simulink model "manipuladores_practica_5"  (R2024b)
settings: Solver=VariableStepAuto  StartTime=0.0  StopTime=10  RelTol=1e-3
settings Model: Creator=alema  LastModifiedBy=alema

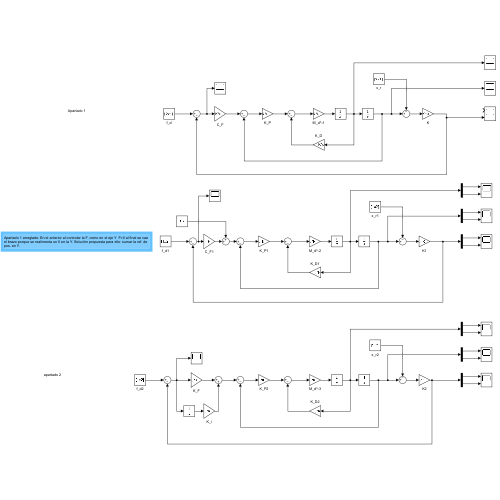
[thumbnail: Simulink's stored preview of the top-level diagram]
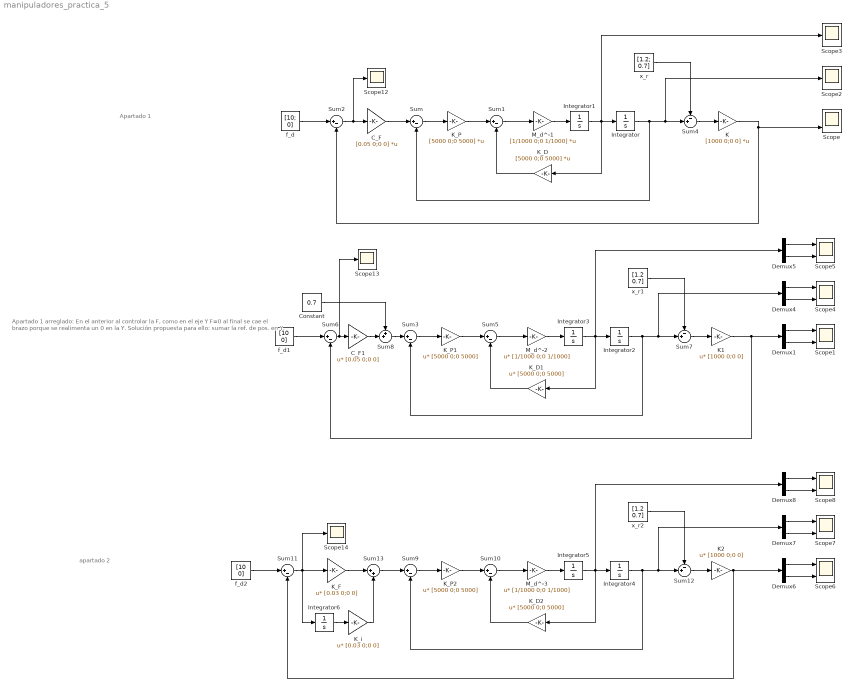
== system manipuladores_practica_5 ==
  note: Apartado 1
  note: Apartado 1 arreglado: En el anterior al controlar la F, como en el eje Y F=0 al final se cae el brazo porque se realimenta un 0 en la Y. Solución propuesta para ello: sumar la ref. de pos. en Y.
  note: apartado 2
  C_F : Gain  Gain=[0.05 0;0 0]  Multiplication=Matrix(K*u)
  C_F1 : Gain  Gain=[0.05 0;0 0]  Multiplication=Matrix(u*K)
  Constant : Constant  Value=0.7
  Demux{1,4..8} (6 alike) : Demux  Outputs=2
  Integrator : Integrator  InitialCondition=[1.3 0.7]
  Integrator1 : Integrator  InitialCondition=[0 0]
  Integrator2 : Integrator  InitialCondition=[1.3 0.7]
  Integrator3 : Integrator  InitialCondition=[0 0]
  Integrator4 : Integrator  InitialCondition=[1.3 0.7]
  Integrator5 : Integrator  InitialCondition=[0 0]
  Integrator6 : Integrator
  K : Gain  Gain=[1000 0;0 0]  Multiplication=Matrix(K*u)
  K1 : Gain  Gain=[1000 0;0 0]  Multiplication=Matrix(u*K)
  K2 : Gain  Gain=[1000 0;0 0]  Multiplication=Matrix(u*K)
  K_D : Gain  Gain=[5000 0;0 5000]  Multiplication=Matrix(K*u)
  K_D1 : Gain  Gain=[5000 0;0 5000]  Multiplication=Matrix(u*K)
  K_D2 : Gain  Gain=[5000 0;0 5000]  Multiplication=Matrix(u*K)
  K_F : Gain  Gain=[0.03 0;0 0]  Multiplication=Matrix(u*K)
  K_P : Gain  Gain=[5000 0;0 5000]  Multiplication=Matrix(K*u)
  K_P1 : Gain  Gain=[5000 0;0 5000]  Multiplication=Matrix(u*K)
  K_P2 : Gain  Gain=[5000 0;0 5000]  Multiplication=Matrix(u*K)
  K_i : Gain  Gain=[0.03 0;0 0]  Multiplication=Matrix(u*K)
  M_d^-1 : Gain  Gain=[1/1000 0;0 1/1000]  Multiplication=Matrix(K*u)
  M_d^-2 : Gain  Gain=[1/1000 0;0 1/1000]  Multiplication=Matrix(u*K)
  M_d^-3 : Gain  Gain=[1/1000 0;0 1/1000]  Multiplication=Matrix(u*K)
  Scope{,1,4..8} (7 alike) : Scope  NumInputPorts=2
  Scope{2..3,12..14} (5 alike) : Scope
  Sum{,1..3,5..6,9..11} (9 alike) : Sum  Inputs=|+-
  Sum12 : Sum  Inputs=-+|
  Sum13 : Sum  Inputs=|++
  Sum4 : Sum  Inputs=-+|
  Sum7 : Sum  Inputs=-+|
  Sum8 : Sum  Inputs=++|
  f_d : Constant  Value=[10; 0]
  f_d1 : Constant  Value=[10 0]
  f_d2 : Constant  Value=[10 0]
  x_r : Constant  Value=[1.2; 0.7]
  x_r1 : Constant  Value=[1.2 0.7]
  x_r2 : Constant  Value=[1.2 0.7]
  wires:
  x_r/1 -> Sum4/1
  Sum4/1 -> K/1
  Integrator/1 -> Sum/2, Scope2/1, Sum4/2
  Sum1/1 -> M_d^-1/1
  M_d^-1/1 -> Integrator1/1
  K_D/1 -> Sum1/2
  K_P/1 -> Sum1/1
  Sum/1 -> K_P/1
  C_F/1 -> Sum/1
  Sum2/1 -> Scope12/1, C_F/1
  f_d/1 -> Sum2/1
  K/1 -> Scope/2, Sum2/2
  Integrator1/1 -> Scope3/1, Integrator/1, K_D/1
  Demux5/2 -> Scope5/2
  Demux4/1 -> Scope4/1
  Demux1/1 -> Scope1/1
  Demux1/2 -> Scope1/2
  K_P1/1 -> Sum5/1
  Integrator2/1 -> Sum3/2, Demux4/1, Sum7/2
  x_r1/1 -> Sum7/1
  Sum6/1 -> Scope13/1, C_F1/1
  K1/1 -> Demux1/1, Sum6/2
  Sum3/1 -> K_P1/1
  f_d1/1 -> Sum6/1
  Integrator3/1 -> Demux5/1, Integrator2/1, K_D1/1
  Demux4/2 -> Scope4/2
  K_D1/1 -> Sum5/2
  Sum7/1 -> K1/1
  Sum5/1 -> M_d^-2/1
  Demux5/1 -> Scope5/1
  M_d^-2/1 -> Integrator3/1
  Sum8/1 -> Sum3/1
  C_F1/1 -> Sum8/2
  Constant/1 -> Sum8/1
  Demux8/2 -> Scope8/2
  Demux7/1 -> Scope7/1
  Demux6/1 -> Scope6/1
  Demux6/2 -> Scope6/2
  K_P2/1 -> Sum10/1
  Integrator4/1 -> Sum9/2, Demux7/1, Sum12/2
  x_r2/1 -> Sum12/1
  K2/1 -> Demux6/1, Sum11/2
  Sum9/1 -> K_P2/1
  f_d2/1 -> Sum11/1
  Integrator5/1 -> Demux8/1, Integrator4/1, K_D2/1
  Demux7/2 -> Scope7/2
  K_D2/1 -> Sum10/2
  Sum12/1 -> K2/1
  Sum10/1 -> M_d^-3/1
  Demux8/1 -> Scope8/1
  M_d^-3/1 -> Integrator5/1
  Sum13/1 -> Sum9/1
  Sum11/1 -> Scope14/1, Integrator6/1, K_F/1
  K_F/1 -> Sum13/1
  K_i/1 -> Sum13/2
  Integrator6/1 -> K_i/1
